simulink model "PI_lead_openloop"  (R2023b)
settings: Solver=ode8  StartTime=0.0  StopTime=20  FixedStep=0.005  RelTol=1e-3
values from neighbouring files (symbols this model uses):
  K = p/z    [lead_vs_leadlag.m]    (also in setup_lead_controller.m)
  p = bodeoptions    [PID_lead_linmod.m]    (also in lead_vs_leadlag.m = 1/(alpha*T); setup_lead_controller.m = 1/(alpha*T))
  z = 1/T    [lead_vs_leadlag.m]    (also in setup_lead_controller.m)
settings Model: Creator=suvo  LastModifiedBy=suvo
settings SolverCC: AlgebraicLoopSolver=TrustRegion
settings DataIOCC: ReturnWorkspaceOutputs=off
settings DebuggingCC: UnconnectedInputMsg=warning  UnconnectedOutputMsg=warning  UnconnectedLineMsg=warning
settings ModelReferenceCC: EnableRefExpFcnMdlSchedulingChecks=on

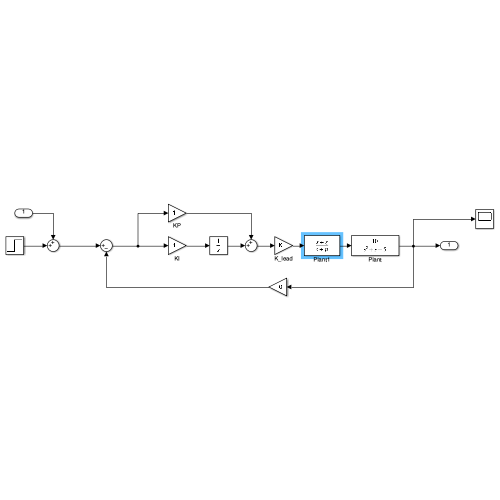
[thumbnail: Simulink's stored preview of the top-level diagram]
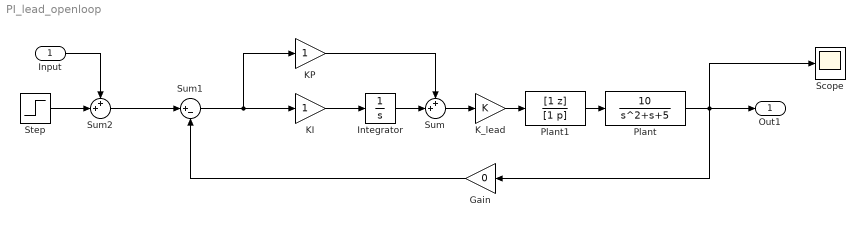
== system PI_lead_openloop ==
  Input : Inport
  Gain : Gain  Gain=0
  Integrator : Integrator
  KI : Gain
  KP : Gain
  K_lead : Gain  Gain=K
  Plant : TransferFcn  Numerator=10  Denominator=[1 1 5]
  Plant1 : TransferFcn  Numerator=[1 z]  Denominator=[1 p]
  Scope : Scope
  Step : Step  SampleTime=0
  Sum : Sum  Inputs=++|
  Sum1 : Sum  Inputs=|+-
  Sum2 : Sum  Inputs=++|
  Out1 : Outport
  wires:
  KI/1 -> Integrator/1
  Sum1/1 -> KP/1, KI/1
  KP/1 -> Sum/1
  Integrator/1 -> Sum/2
  Plant/1 -> Out1/1, Gain/1, Scope/1
  Sum/1 -> K_lead/1
  Gain/1 -> Sum1/2
  Step/1 -> Sum2/2
  Input/1 -> Sum2/1
  Sum2/1 -> Sum1/1
  Plant1/1 -> Plant/1
  K_lead/1 -> Plant1/1
